simulink model "TR_Module_Datasheet"  (R2025b)
settings: Solver=FixedStepDiscrete  StartTime=0.0  StopTime=inf  RelTol=1e-3
InitFcn:
  | fc = 2.4e9;
model workspace (MATLAB code in the model file):
  | Fc = 2.4e9;
  | N = 8;
  | load('dualPolarizedAntennaAnalysis.mat','dualPolarizedAntenna');
  | inAM  = [0.1 1  2  3   4   5]';
  | outAM = [5 50 85 110 115 120]';
  | outPM = [0 1  2  10  20  50]';
  | ampmTablePA = [10*log10(inAM)+30 ...
  |     10*log10(outAM)+30 ...
  |     outPM];
undefined symbols (not defined in the file or in its folder): rational, S, sparameters
libraries: simrfV2elements x10, dspstat3 x4, simrfV2util1 x3, simrfV2junction1 x3, rfBudgetAnalyzer_lib x1
settings Model: Creator=The MathWorks, Inc.  LastModifiedBy=galberti
settings SolverCC: MaxZcPerStep=1.0
settings DataIOCC: SaveOutput=off  SignalLogging=off  DSMLogging=off  SaveTime=off  ReturnWorkspaceOutputs=off
settings ModelReferenceCC: EnableRefExpFcnMdlSchedulingChecks=on
settings RTWCC: GPUComputeCapability=3.5  DLArmComputeVersion=19.05

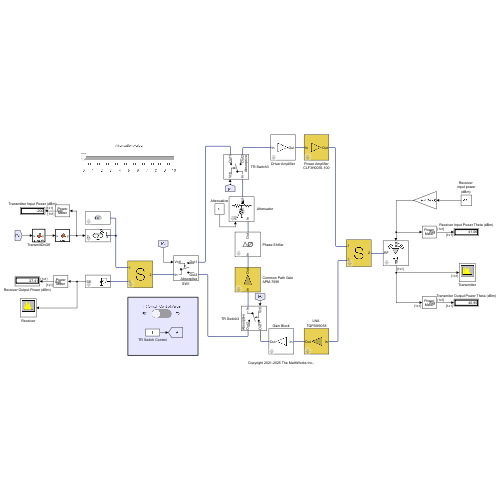
[thumbnail: Simulink's stored preview of the top-level diagram]
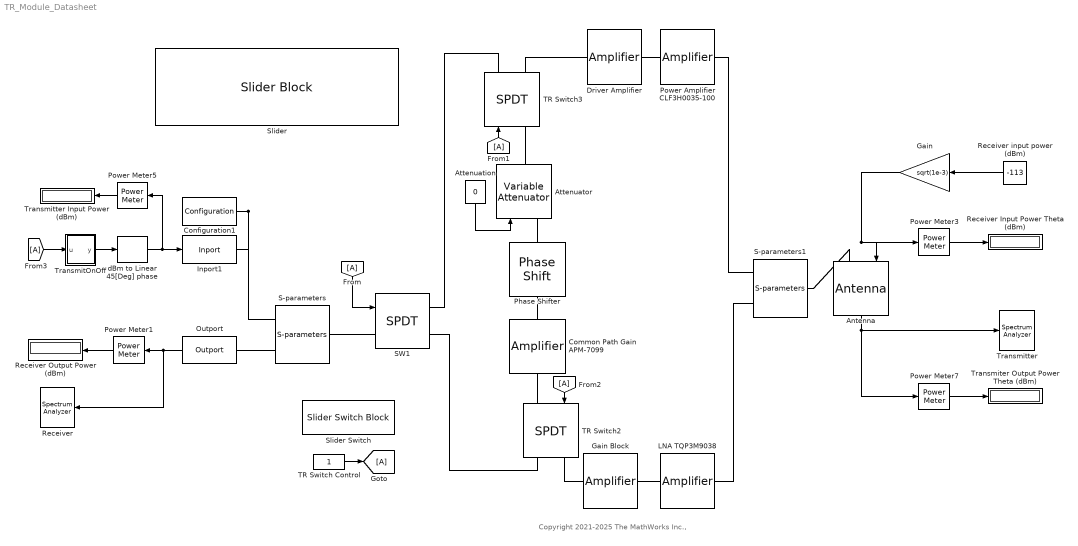
== system TR_Module_Datasheet ==
  note: Copyright 2021-2025 The MathWorks Inc.,
  " Attenuator" : simrfV2elements/Variable Attenuator  classname=varattenuator  Attmin=0.01  Attmax=10  Zin=50  Zout=50  AddNoise=on  InternalGrounding=on
  Antenna : simrfV2elements/Antenna  CacheLevel=0  AntennaSource=Isotropic radiator  PrevAppliedAntSource=Isotropic radiator  Gr=0 dBi  Zin=50  AntennaObj=antObj  InputIncWave=on  OutputRadWave=on  CarrierFreqInc=fc Hz  rArr=[180 0] deg  CarrierFreqRad=fc Hz  rDep=[0 0] deg  AddNoise=on  InternalGrounding=on  SparamRepresentationImp=Time domain  FitTolImp=-40  AutoImpulseLengthImp=on  ImpulseLengthImp=1e-10 s
  Attenuation : Constant  Value=0
  Common Path Gain APM-7099 : simrfV2elements/Amplifier  classname=amplifier  DataSource=Data file  File=unitygain.s2p  isNetworkObj=off  NetworkObject=sparameters('default.s2p')  Paramtype=S-parameters  Sparam=[0 0;1 0]  SparamFreq=1e9 Hz  SparamZ0=50  isRationalObj=off  RationalObject=rational('default.s2p')  Residues=0  Poles=0  DF={0 0; 1 0}  Source_linear_gain=Available power gain  linear_gain=14 dB  AmAmAmPmTable=[-25,5,-1;-10,20,-2;0,27,5;5,28,12]  Zin=50  Zout=50  Source_Poly=Odd order  Poly_Coeffs=[0 1]  IPType=Output  IP2=inf dBm  IP3=38 dBm  P1dB=27 dBm  Psat=inf dBm  Gcomp=0 dBm  InternalGrounding=on  SourceFreq=Extracted from data source  PlotFreq=[1e9:1e6:3e9] Hz  PlotType=X-Y plane  YParam1=S(1,1)  YFormat1=Magnitude (dB)  YParam2=None  YFormat2=Magnitude (dB)  YOption=Linear  XOption=Linear  SparamRepresentation=Time domain  FitTol=-40  FitOpt=Fit individually  MaxPoles=48  AutoImpulseLength=on  ImpulseLength=1e-10 s  MagModeling=off  AddNoise=on  NoiseType=Noise figure  NoiseDist=White  NF=5  MinNF=0  Gopt=0  RN=0  CarrierFreq=0 Hz  NoiseAutoImpulseLength=on  NoiseImpulseLength=1e-10 s  ConstS21NL=off  OpFreq=1 GHz  SetOpFreqAsMaxS21=on
  Configuration1 : simrfV2util1/Configuration  AutoFreq=off  Tones=fc Hz  Harmonics=3  NormalizeCarrierPower=on  SolverType=Auto  UseCCode=on  StepSize=1e-5 s  AddNoise=on  defaultRNG=on  Seed=0  Temperature=290.0 K  SolverDelFlag=0  AbsTol=1e-6  RelTol=1e-3  MaxIter=10  ErrorEstimationType=2-norm over all variables  EnableInterpFilter=on  HiddenFIRfilterControllerParam=off  SmallSignalApprox=off  AllSimFreqs=on  SimFreqs=[] Hz  SimFreqsInternal=[]  SamplesPerFrame=1
  Driver Amplifier : simrfV2elements/Amplifier  classname=amplifier  DataSource=Data file  File=unitygain.s2p  isNetworkObj=off  NetworkObject=sparameters('default.s2p')  Paramtype=S-parameters  Sparam=[0 0;1 0]  SparamFreq=1e9 Hz  SparamZ0=50  isRationalObj=off  RationalObject=rational('default.s2p')  Residues=0  Poles=0  DF={0 0; 1 0}  Source_linear_gain=Available power gain  linear_gain=25 dB  AmAmAmPmTable=[-25,5,-1;-10,20,-2;0,27,5;5,28,12]  Zin=50  Zout=50  Source_Poly=Even and odd order  Poly_Coeffs=[0 1]  IPType=Output  IP2=inf dBm  IP3=inf dBm  P1dB=inf dBm  Psat=inf dBm  Gcomp=inf dBm  InternalGrounding=on  SourceFreq=Extracted from data source  PlotFreq=[1e9:1e6:3e9] Hz  PlotType=X-Y plane  YParam1=S(1,1)  YFormat1=Magnitude (dB)  YParam2=None  YFormat2=Magnitude (dB)  YOption=Linear  XOption=Linear  SparamRepresentation=Time domain  FitTol=-40  FitOpt=Fit individually  MaxPoles=48  AutoImpulseLength=on  ImpulseLength=1e-10 s  MagModeling=off  AddNoise=off  NoiseType=Noise figure  NoiseDist=White  NF=0  MinNF=0  Gopt=0  RN=0  CarrierFreq=0 Hz  NoiseAutoImpulseLength=on  NoiseImpulseLength=1e-10 s  ConstS21NL=off  OpFreq=1 GHz  SetOpFreqAsMaxS21=on
  From{,1..3} (4 alike) : From
  Gain : Gain  Gain=sqrt(1e-3)
  Gain Block : simrfV2elements/Amplifier  classname=amplifier  DataSource=Data file  File=unitygain.s2p  isNetworkObj=off  NetworkObject=sparameters('default.s2p')  Paramtype=S-parameters  Sparam=[0 0;1 0]  SparamFreq=1e9 Hz  SparamZ0=50  isRationalObj=off  RationalObject=rational('default.s2p')  Residues=0  Poles=0  DF={0 0; 1 0}  Source_linear_gain=Available power gain  linear_gain=15 dB  AmAmAmPmTable=[-25,5,-1;-10,20,-2;0,27,5;5,28,12]  Zin=50  Zout=50  Source_Poly=Even and odd order  Poly_Coeffs=[0 1]  IPType=Output  IP2=inf dBm  IP3=inf dBm  P1dB=inf dBm  Psat=inf dBm  Gcomp=inf dBm  InternalGrounding=on  SourceFreq=Extracted from data source  PlotFreq=[1e9:1e6:3e9] Hz  PlotType=X-Y plane  YParam1=S(1,1)  YFormat1=Magnitude (dB)  YParam2=None  YFormat2=Magnitude (dB)  YOption=Linear  XOption=Linear  SparamRepresentation=Time domain  FitTol=-40  FitOpt=Fit individually  MaxPoles=48  AutoImpulseLength=on  ImpulseLength=1e-10 s  MagModeling=off  AddNoise=off  NoiseType=Noise figure  NoiseDist=White  NF=0  MinNF=0  Gopt=0  RN=0  CarrierFreq=0 Hz  NoiseAutoImpulseLength=on  NoiseImpulseLength=1e-10 s  ConstS21NL=off  OpFreq=1 GHz  SetOpFreqAsMaxS21=on
  Goto : Goto
  Inport1 : simrfV2util1/Inport  SimulinkInputSignalType=Power  CarrierFreq=fc Hz  ZS=50  UseSqWave=off  NumCoeff=10  Bias=0  DutyCyc=50  InternalGrounding=on
  LNA TQP3M9038 : simrfV2elements/Amplifier  classname=amplifier  DataSource=Data file  File=TQP3M9038.s2p  isNetworkObj=off  NetworkObject=sparameters('default.s2p')  Paramtype=S-parameters  Sparam=[0 0;1 0]  SparamFreq=1e9 Hz  SparamZ0=50  isRationalObj=off  RationalObject=rational('default.s2p')  Residues=0  Poles=0  DF={0 0; 1 0}  Source_linear_gain=Data source  linear_gain=17 dB  AmAmAmPmTable=[-25,5,-1;-10,20,-2;0,27,5;5,28,12]  Zin=50  Zout=50  Source_Poly=Even and odd order  Poly_Coeffs=[0 1]  IPType=Output  IP2=inf dBm  IP3=40 dBm  P1dB=inf dBm  Psat=inf dBm  Gcomp=inf dBm  InternalGrounding=on  SourceFreq=Extracted from data source  PlotFreq=[1e9:1e6:3e9] Hz  PlotType=X-Y plane  YParam1=S(2,1)  YFormat1=Magnitude (dB)  YParam2=None  YFormat2=Magnitude (dB)  YOption=Linear  XOption=Linear  SparamRepresentation=Time domain  FitTol=-40  FitOpt=Fit individually  MaxPoles=48  AutoImpulseLength=on  ImpulseLength=1e-10 s  MagModeling=off  AddNoise=on  NoiseType=Noise figure  NoiseDist=White  NF=2  MinNF=0  Gopt=0  RN=0  CarrierFreq=0 Hz  NoiseAutoImpulseLength=on  NoiseImpulseLength=1e-10 s  ConstS21NL=off  OpFreq=Fc Hz  SetOpFreqAsMaxS21=on
  Outport : simrfV2util1/Outport  SensorType=Power  OutputFormat=Complex Baseband  CarrierFreq=fc Hz  ZL=50  InternalGrounding=on  StepSize=1e-6 s  AutoStep=on  HalfPolyphaseLength=12
  Phase Shifter : simrfV2elements/Phase Shift  PhaseShift=90 deg  InternalGrounding=on  PCBConvertable=on  PCBObjDesign={'design(phaseShifter,<DesignFreq>,''PhaseShift'',convert2Deg(<PhaseShift>,<PhaseShift_unit>))'}  PCBObjAllowed={{'phaseShifter'}}  PCBObjReroute={cell(1,0)}
  Power Amplifier CLF3H0035-100 : simrfV2elements/Amplifier  classname=amplifier  DataSource=Data file  File=unitygain.s2p  isNetworkObj=off  NetworkObject=sparameters('default.s2p')  Paramtype=S-parameters  Sparam=[0 0;1 0]  SparamFreq=1e9 Hz  SparamZ0=50  isRationalObj=off  RationalObject=rational('default.s2p')  Residues=0  Poles=0  DF={0 0; 1 0}  Source_linear_gain=AM/AM-AM/PM table  linear_gain=15 dB  AmAmAmPmTable=ampmTablePA  Zin=50  Zout=50  Source_Poly=Odd order  Poly_Coeffs=[0 1]  IPType=Output  IP2=inf dBm  IP3=inf dBm  P1dB=inf %51 dBm  Psat=inf dBm  Gcomp=inf dBm  InternalGrounding=on  SourceFreq=Extracted from data source  PlotFreq=[1e9:1e6:3e9] Hz  PlotType=X-Y plane  YParam1=S(1,1)  YFormat1=Magnitude (dB)  YParam2=None  YFormat2=Magnitude (dB)  YOption=Linear  XOption=Linear  SparamRepresentation=Time domain  FitTol=-40  FitOpt=Fit individually  MaxPoles=48  AutoImpulseLength=on  ImpulseLength=1e-10 s  MagModeling=off  AddNoise=off  NoiseType=Noise figure  NoiseDist=White  NF=0  MinNF=0  Gopt=0  RN=0  CarrierFreq=0 Hz  NoiseAutoImpulseLength=on  NoiseImpulseLength=1e-10 s  ConstS21NL=off  OpFreq=1 GHz  SetOpFreqAsMaxS21=on
  Power Meter{1,3,5,7} (4 alike) : dspstat3/Power Meter  Measurement=Average power  ReferenceLoad=1  OutputPowerUnits=dBm  WindowLength=256  OverlapLength=255  AllowArbitraryInputLength=off  ComputeCCDF=off  PowerRange=50  PowerResolution=0.1  CCDFOutput=Relative power (dB above average power)  ProbabilityVector=[ 10; 1; 0.1; 0.01; 0.001; 0.0001 ]  RelativePowerVector=[ 0; 3; 6; 9; 12 ]  ResetPort=off  SimulateUsing=Code generation
      settings: LibrarySourceBlock=commutil2/Power Meter
  Receiver : SpectrumAnalyzer  WindowPosition=[570.000000,14.000000,487.000000,351.000000,]  Visible=on  ScopeFrameLocation=window  Method=Welch  Span=100000000  StartFrequency=-50000000  StopFrequency=50000000  AveragingMethod=Exponential  ForgettingFactor=0.5  YLimits=[-53.801 33.3772]  ColorLimits=[-80 20]  ShowLegend=on  SelectedToolstripTab=spectrumAnalyzerToolstrip.measurementsTab  AllowFFTLengthLessThanSamplesPerUpdate=on
  "Receiver input power (dBm) " : Constant  Value=-113
  Receiver Input Power Theta (dBm) : Display
  Receiver Output Power (dBm) : Display
  S-parameters : simrfV2elements/S-parameters  classname=sparam_element  DataSource=Data file  File=TX_Circulator.s3p  isNetworkObj=on  NetworkObject=cir  Paramtype=S-parameters  Sparam=[0 0;1 0]  SparamFreq=1e9 Hz  SparamZ0=50  isRationalObj=off  RationalObject=rational('default.s2p')  Residues=0  Poles=0  DF={0 0; 1 0}  FitOpt=Share all poles  FitTol=-40  MaxPoles=48  SourceFreq=Extracted from data source  PlotFreq=[1e9:1e6:3e9] Hz  PlotType=X-Y plane  YParam1=S(2,1)  YFormat1=Magnitude (dB)  YParam2=None  YFormat2=Magnitude (dB)  YOption=Linear  XOption=Linear  AddNoise=off  InternalGrounding=on  SparamRepresentation=Time domain  AutoImpulseLength=on  ImpulseLength=1e-10 s  MagModeling=off  CacheLevel=0
  S-parameters1 : simrfV2elements/S-parameters  classname=sparam_element  DataSource=Data file  File=TX_Circulator.s3p  isNetworkObj=on  NetworkObject=cir  Paramtype=S-parameters  Sparam=[0 0;1 0]  SparamFreq=1e9 Hz  SparamZ0=50  isRationalObj=off  RationalObject=rational('default.s2p')  Residues=0  Poles=0  DF={0 0; 1 0}  FitOpt=Share all poles  FitTol=-40  MaxPoles=48  SourceFreq=Extracted from data source  PlotFreq=[1e9:1e6:3e9] Hz  PlotType=X-Y plane  YParam1=S(1,1)  YFormat1=Magnitude (dB)  YParam2=None  YFormat2=Magnitude (dB)  YOption=Linear  XOption=Linear  AddNoise=off  InternalGrounding=on  SparamRepresentation=Time domain  AutoImpulseLength=on  ImpulseLength=1e-10 s  MagModeling=off  CacheLevel=0
  SW1 : simrfV2junction1/SPDT  classname=spdt  SwitchType=switchSPDT  Vthres=2.5 V  CharType=Insertion loss  Ron=10 Ohm  Roff=1e6 Ohm  Iloss=0.01  Iiso=100  LoadType=Absorptive  Z0=50 Ohm  InternalGrounding=on
  Slider : SliderBlock  ScaleMax=10  TickInterval=1
  Slider Switch : SliderSwitchBlock
  TR Switch Control : Constant
  TR Switch2 : simrfV2junction1/SPDT  classname=spdt  SwitchType=switchSPDT  Vthres=2.5 V  CharType=Insertion loss  Ron=10 Ohm  Roff=1e6 Ohm  Iloss=0.01  Iiso=100  LoadType=Absorptive  Z0=50 Ohm  InternalGrounding=on
  TR Switch3 : simrfV2junction1/SPDT  classname=spdt  SwitchType=switchSPDT  Vthres=2.5 V  CharType=Insertion loss  Ron=10 Ohm  Roff=1e6 Ohm  Iloss=0.01  Iiso=100  LoadType=Absorptive  Z0=50 Ohm  InternalGrounding=on
  TransmitOnOff : MATLAB Function  TreatAsAtomicUnit=on
  Transmiter Output Power Theta (dBm) : Display
  Transmitter : SpectrumAnalyzer  WindowPosition=[67.000000,-46.000000,496.000000,411.000000,]  Visible=on  ScopeFrameLocation=window  Method=Welch  Span=80000000  StartFrequency=-40000000  StopFrequency=40000000  AveragingMethod=Exponential  ForgettingFactor=0.6  YLimits=[-31.9014 50.9554]  ColorLimits=[-80 20]  ShowLegend=on  SelectedToolstripTab=spectrumAnalyzerToolstrip.measurementsTab  AllowFFTLengthLessThanSamplesPerUpdate=on
  Transmitter Input Power (dBm) : Display
  dBm to Linear 45[Deg] phase : rfBudgetAnalyzer_lib/dBm to Linear 45[Deg] phase  SystemSampleTime=-1  VariantActivationTime=update diagram  EmptyChoice=off  PassThrough=off  PassThroughVariantControl=(default)  EmptyChoiceVariantControl=(default)  AllowFlexibleInterface=on  Latency=0  AutoFrameSizeCalculation=off
  wires:
  Attenuation/1 -> " Attenuator"/1
  Outport/1 -> Power Meter1/1, Receiver/1
  Power Meter1/1 -> Receiver Output Power (dBm)/1
  From3/1 -> TransmitOnOff/1(u)
  Power Meter5/1 -> Transmitter Input Power (dBm)/1
  Antenna/1 -> Power Meter7/1, Transmitter/1
  Power Meter7/1 -> Transmiter Output Power Theta (dBm)/1
  "Receiver input power (dBm) "/1 -> Gain/1
  Power Meter3/1 -> Receiver Input Power Theta (dBm)/1
  dBm to Linear 45[Deg] phase/1 -> Inport1/1, Power Meter5/1
  TR Switch Control/1 -> Goto/1
  From/1 -> SW1/1
  From1/1 -> TR Switch3/1
  From2/1 -> TR Switch2/1
  TransmitOnOff/1(y) -> dBm to Linear 45[Deg] phase/1
  Gain/1 -> Antenna/1, Power Meter3/1
  connections:
  Power Amplifier CLF3H0035-100/LConn1 -- Driver Amplifier/RConn1
  S-parameters/RConn1 -- SW1/LConn1
  LNA TQP3M9038/RConn1 -- Gain Block/LConn1
  Phase Shifter/RConn1 -- " Attenuator"/LConn1
  TR Switch3/LConn1 -- " Attenuator"/RConn1
  Common Path Gain APM-7099/RConn1 -- Phase Shifter/LConn1
  Common Path Gain APM-7099/LConn1 -- TR Switch2/LConn1
  SW1/RConn2 -- TR Switch2/RConn2
  TR Switch2/RConn1 -- Gain Block/RConn1
  SW1/RConn1 -- TR Switch3/RConn1
  TR Switch3/RConn2 -- Driver Amplifier/LConn1
  S-parameters1/LConn1 -- Power Amplifier CLF3H0035-100/RConn1
  Configuration1/LConn1 -- S-parameters/LConn1 -- Inport1/RConn1
  S-parameters1/LConn2 -- LNA TQP3M9038/LConn1
  S-parameters/LConn2 -- Outport/LConn1
  Antenna/LConn1 -- S-parameters1/RConn1

== matlab function TR_Module_Datasheet/TransmitOnOff ==
  data: u input; y output
function y = OnOff(u)
if u<2.5
    y = -200; % do not transmit (receive)
else
    y = 3; %transmit
end
